simulink model "ex_problem_default_configuration"  (R2024a)
settings: Solver=VariableStepAuto  StartTime=0.0  StopTime=100  FixedStep=1  RelTol=1e-6
libraries: simulink x1
settings Model: Creator=j.morlier  LastModifiedBy=a.brugnoli
settings SolverCC: AlgebraicLoopSolver=TrustRegion
settings DataIOCC: ReturnWorkspaceOutputs=off
settings DebuggingCC: UnconnectedInputMsg=warning  UnconnectedOutputMsg=warning  UnconnectedLineMsg=warning  ArithmeticOperatorsInVariantConditions=warning
settings ModelReferenceCC: EnableRefExpFcnMdlSchedulingChecks=on
settings SFSimCC: SimUseLocalCustomCode=off  CustomCodeUndefinedFunction=UseInterfaceOnly
settings RTWCC: RTWUseLocalCustomCode=off  GPUComputeCapability=3.5

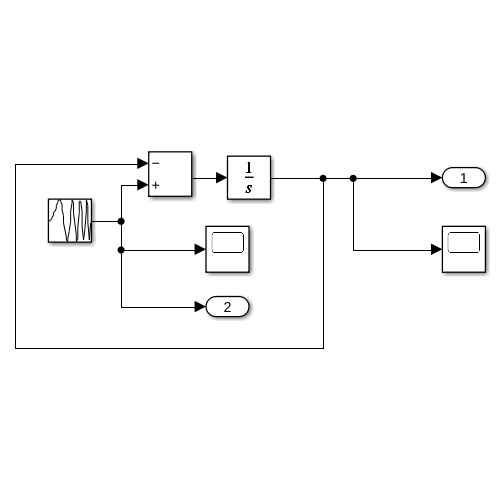
[thumbnail: Simulink's stored preview of the top-level diagram]
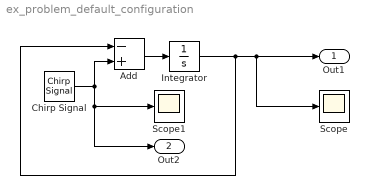
== system ex_problem_default_configuration ==
  Add : Sum  Inputs=-+
  Chirp Signal : simulink/Sources/Chirp Signal  f1=0.1  T=100  f2=1
  Integrator : Integrator
  Scope : Scope
  Scope1 : Scope
  Out1 : Outport
  Out2 : Outport  Port=2
  wires:
  Add/1 -> Integrator/1
  Integrator/1 -> Scope/1, Out1/1, Add/1
  Chirp Signal/1 -> Add/2, Out2/1, Scope1/1
